simulink model "RLC_Serie_PassaFaixa"  (R2020a)
settings: Solver=ode23tb  StartTime=0.0  StopTime=10  MaxStep=1e-4  RelTol=1e-3  EnableMultiTasking=on
undefined symbols (not defined in the file or in its folder): C, L, R
libraries: powerlib x7
settings Model: Creator=renat  LastModifiedBy=Djalma_Win10
settings DataIOCC: ReturnWorkspaceOutputs=off
settings OptimizationCC: LifeSpan=inf
settings DebuggingCC: SFUnexpectedBacktrackingDiag=warning  SFNoUnconditionalDefaultTransitionDiag=warning  ArithmeticOperatorsInVariantConditions=warning
settings SFSimCC: SimUseLocalCustomCode=off  CustomCodeUndefinedFunction=UseInterfaceOnly
settings RTWCC: RTWUseLocalCustomCode=off
settings CodeAppCC: StateflowObjectComments=on
settings GRTTargetCC: TargetLangStandard=C89/C90 (ANSI)
settings ConfigComp: CovMetricSettings=dw  CovHtmlReporting=on  CovSaveCumulativeToWorkspaceVar=on  CovSaveSingleToWorkspaceVar=on  CovExternalEMLEnable=off
settings SimscapeCC: SimscapeNormalizeSystem=off

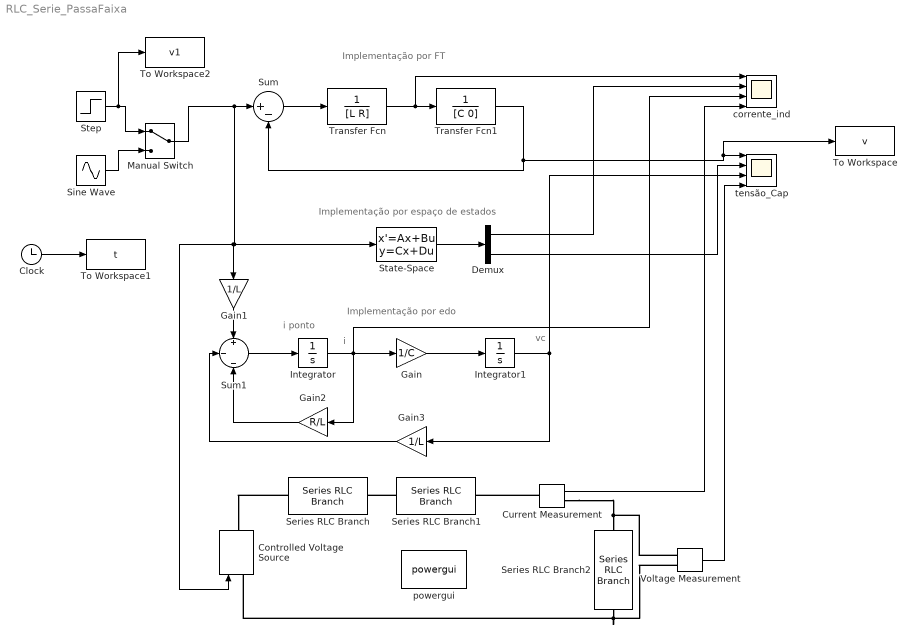
== system RLC_Serie_PassaFaixa ==
  note: vc
  note: i
  note: i ponto
  note: Implementação por edo
  note: Implementação por espaço de estados
  note: Implementação por FT
  Clock : Clock
      settings: Decimation=5
  Controlled Voltage Source : powerlib/Electrical Sources/Controlled Voltage Source  Initialize=on  Source_Type=AC  Amplitude=0  Phase=0  Frequency=0  Measurements=None
  Current Measurement : powerlib/Measurements/Current Measurement  PhasorSimulation=off  OutputType=Complex  PSBequivalent=0
  Demux : Demux  Outputs=2
  Gain : Gain  Gain=1/C
  Gain1 : Gain  Gain=1/L
  Gain2 : Gain  Gain=R/L
  Gain3 : Gain  Gain=1/L
  Integrator : Integrator
  Integrator1 : Integrator
  Manual Switch : ManualSwitch
  Series RLC Branch : powerlib/Elements/Series RLC Branch  LConnTagsString=__new0  RConnTagsString=__new0  BranchType=R  Resistance=R  Inductance=1e-3  SetiL0=off  InitialCurrent=0  Capacitance=1e-6  Setx0=off  InitialVoltage=0  Measurements=None
  Series RLC Branch1 : powerlib/Elements/Series RLC Branch  LConnTagsString=__new0  RConnTagsString=__new0  BranchType=L  Resistance=R  Inductance=L  SetiL0=off  InitialCurrent=0  Capacitance=1e-6  Setx0=off  InitialVoltage=0  Measurements=None
  Series RLC Branch2 : powerlib/Elements/Series RLC Branch  LConnTagsString=__new0  RConnTagsString=__new0  BranchType=C  Resistance=R  Inductance=L  SetiL0=off  InitialCurrent=0  Capacitance=C  Setx0=off  InitialVoltage=0  Measurements=None
  Sine Wave : Sin  Amplitude=10*sqrt(2)  Frequency=2*pi*100  SampleTime=0
  State-Space : StateSpace  A=[-R/L -1/L; 1/C 0]  B=[1/L; 0]  C=[1 0; 0 1]  D=[0; 0]  InitialCondition=0
  Step : Step  Time=0  After=10  SampleTime=0
  Sum : Sum  Inputs=|+-
  Sum1 : Sum  Inputs=+|-|-
  To Workspace : ToWorkspace  VariableName=v  SampleTime=-1
  To Workspace1 : ToWorkspace  VariableName=t  SampleTime=-1
  To Workspace2 : ToWorkspace  VariableName=v1  SampleTime=-1
  Transfer Fcn : TransferFcn  Denominator=[L R]
  Transfer Fcn1 : TransferFcn  Denominator=[C 0]
  Voltage Measurement : powerlib/Measurements/Voltage Measurement  PhasorSimulation=off  OutputType=Complex  PSBequivalent=0
  corrente_ind : Scope  NumInputPorts=4
  powergui : powerlib/powergui  Priority=1  SimulationMode=Continuous  SampleTime=50e-6  frequency=60  Iterations=50  frequencyindice=0  Pbase=100e6  ErrMax=1e-4  UnitsV=kV  UnitsW=MW  buscounter=0  FunctionMessages=off  echomessages=off  EnableUseOfTLC=off  CurrentSourceSwitches=off  DisableSnubberDevices=off  DisableRonSwitches=off  DisableVfSwitches=off  DisplayEquations=off  AutomaticDiscreteSolvers=off  SolverType=Tustin/Backward Euler (TBE)  Interpol=off  ExternalGateDelay=off  methode=off  Ts=10  x0status=blocks  SPID=off  SwTol=0  HookPort=off  NonlinearTolerance=1e-4  nMaxIteration=100  ContinueOnMaxIteration=off  RestoreLinks=warning  ResistiveCurrentMeasurement=off  Frange=[0:2:500]  Ylog=off  Xlog=on  ShowGrid=off  save=off  variable=ZData  structure=0  ZoomFFT=off  StartTime=0.0  cycles=1  DisplayStyle=1  fundamental=60  FreqAxis=off  MaxFrequency=1000  frequencyindicesteady=1  RmsSteady=1  display=off
  tensão_Cap : Scope  NumInputPorts=4
  wires:
  Manual Switch/1 -> Controlled Voltage Source/1, Gain1/1, State-Space/1, Sum/1
  Sum/1 -> Transfer Fcn/1
  Transfer Fcn/1 -> corrente_ind/1, Transfer Fcn1/1
  Transfer Fcn1/1 -> To Workspace/1, tensão_Cap/1, Sum/2
  State-Space/1 -> Demux/1
  Demux/1 -> corrente_ind/2
  Demux/2 -> tensão_Cap/2
  Sum1/1 -> Integrator/1
  Gain1/1 -> Sum1/1
  Integrator/1 -> corrente_ind/3, Gain/1, Gain2/1
  Gain2/1 -> Sum1/3
  Gain3/1 -> Sum1/2
  Integrator1/1 -> Gain3/1, tensão_Cap/3
  Gain/1 -> Integrator1/1
  Current Measurement/1 -> corrente_ind/4
  Voltage Measurement/1 -> tensão_Cap/4
  Step/1 -> To Workspace2/1, Manual Switch/1
  Sine Wave/1 -> Manual Switch/2
  Clock/1 -> To Workspace1/1
  connections:
  Series RLC Branch1/LConn1 -- Series RLC Branch/RConn1
  Current Measurement/LConn1 -- Series RLC Branch1/RConn1
  Series RLC Branch/LConn1 -- Controlled Voltage Source/RConn1
  Current Measurement/RConn1 -- Voltage Measurement/LConn1 -- Series RLC Branch2/LConn1
  Series RLC Branch2/RConn1 -- Controlled Voltage Source/LConn1 -- Voltage Measurement/LConn2
